simulink model "vssSimulation"  (R2023a)
settings: Solver=FixedStepAuto  StartTime=0.0  StopTime=5  FixedStep=0.002  RelTol=1e-3
settings Model: Creator=Dell Precision  LastModifiedBy=Dell Precision

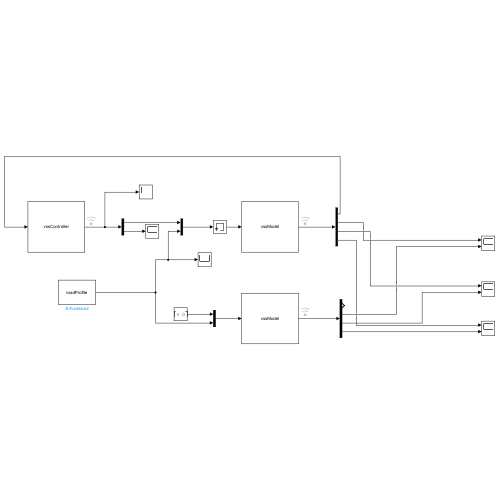
[thumbnail: Simulink's stored preview of the top-level diagram]
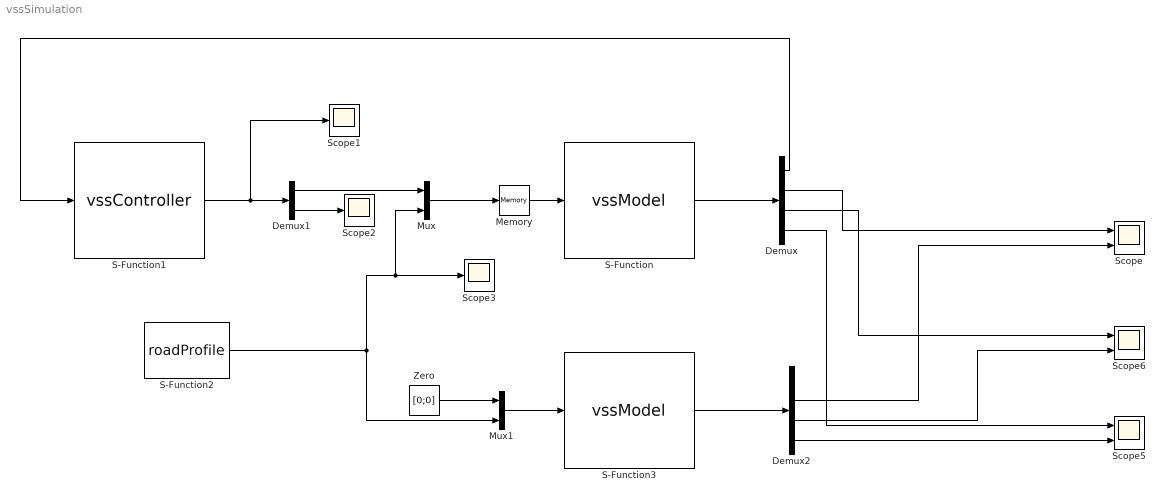
== system vssSimulation ==
  Demux : Demux  Outputs=[8;2;2;2]
  Demux1 : Demux  Outputs=[2;1]
  Demux2 : Demux  Outputs=[8;2;2;2]
  Memory : Memory
  Mux : Mux  Inputs=2
  Mux1 : Mux  Inputs=2
  S-Function : S-Function  FunctionName=vssModel  SFunctionDeploymentMode=off  EnableBusSupport=off
  S-Function1 : S-Function  FunctionName=vssController  SFunctionDeploymentMode=off  EnableBusSupport=off
  S-Function2 : S-Function  FunctionName=roadProfile  SFunctionDeploymentMode=off  EnableBusSupport=off
  S-Function3 : S-Function  FunctionName=vssModel  SFunctionDeploymentMode=off  EnableBusSupport=off
  Scope : Scope  NumInputPorts=2
  Scope1 : Scope
  Scope2 : Scope
  Scope3 : Scope
  Scope5 : Scope  NumInputPorts=2
  Scope6 : Scope  NumInputPorts=2
  Zero : Constant  Value=[0;0]  OutDataTypeStr=Inherit: Inherit via back propagation
  wires:
  Mux/1 -> Memory/1
  S-Function1/1 -> Scope1/1, Demux1/1
  S-Function2/1 -> Scope3/1, Mux/2, Mux1/2
  S-Function/1 -> Demux/1
  Demux/1 -> S-Function1/1
  Demux/2 -> Scope/1
  Memory/1 -> S-Function/1
  Demux1/1 -> Mux/1
  Demux1/2 -> Scope2/1
  Mux1/1 -> S-Function3/1
  Zero/1 -> Mux1/1
  S-Function3/1 -> Demux2/1
  Demux/3 -> Scope6/1
  Demux2/2 -> Scope/2
  Demux2/3 -> Scope6/2
  Demux/4 -> Scope5/1
  Demux2/4 -> Scope5/2
